simulink model "m100_ControlSystem"  (R2022a)
settings: Solver=VariableStepAuto  StartTime=0.0  StopTime=10.0  RelTol=1e-3
libraries: simulink x1
settings Model: Creator=Admin  LastModifiedBy=Admin
settings DataIOCC: Refine=10

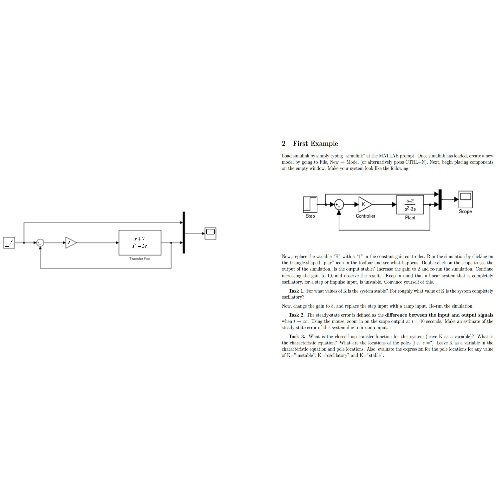
[thumbnail: Simulink's stored preview of the top-level diagram]
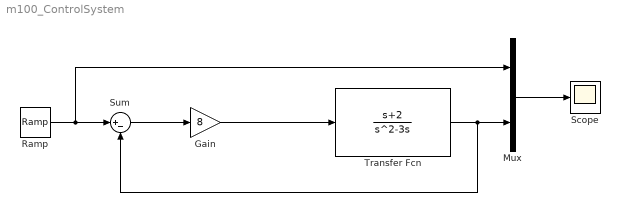
== system m100_ControlSystem ==
  Gain : Gain  Gain=8
  Mux : Mux  Inputs=2
  Ramp : simulink/Sources/Ramp  slope=1  start=0  InitialOutput=0
  Scope : Scope
  Sum : Sum  Inputs=|+-
  Transfer Fcn : TransferFcn  Numerator=[1 2]  Denominator=[1 -3 0]
  wires:
  Transfer Fcn/1 -> Sum/2, Mux/2
  Ramp/1 -> Mux/1, Sum/1
  Sum/1 -> Gain/1
  Gain/1 -> Transfer Fcn/1
  Mux/1 -> Scope/1
